simulink model "Lab2Task1"  (R2016a)
settings: Solver=VariableStepAuto  StartTime=0.0  StopTime=10.0  RelTol=1e-3
settings Model: Creator=Thomas  LastModifiedBy=Thomas

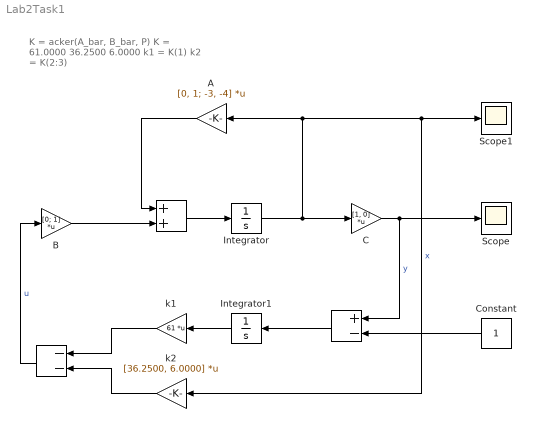
== system Lab2Task1 ==
  note: K = acker(A_bar, B_bar, P)
      | K =   61.0000   36.2500    6.0000
      | k1 = K(1)
      | k2 = K(2:3)
  " " : Sum  Inputs=+-
  "  " : Sum  Inputs=--
  "   " : Sum
  A : Gain  Gain=[0, 1; -3, -4]  Multiplication=Matrix(K*u)
  B : Gain  Gain=[0; 1]  Multiplication=Matrix(K*u)
  C : Gain  Gain=[1, 0]  Multiplication=Matrix(K*u)
  Constant : Constant
  Integrator : Integrator  InitialCondition=[0.3;0.4]
  Integrator1 : Integrator
  Scope : Scope
  Scope1 : Scope
  k1 : Gain  Gain=61  Multiplication=Matrix(K*u)
  k2 : Gain  Gain=[36.2500, 6.0000]  Multiplication=Matrix(K*u)
  wires:
  "   "/1 -> Integrator/1
  A/1 -> "   "/1
  B/1 -> "   "/2
  Integrator/1 -> A/1, k2/1, Scope1/1, C/1  "x"
  C/1 -> " "/1, Scope/1  "y"
  " "/1 -> Integrator1/1
  Integrator1/1 -> k1/1
  k1/1 -> "  "/1
  "  "/1 -> B/1  "u"
  k2/1 -> "  "/2
  Constant/1 -> " "/2
